simulink model "L_I"  (R2013a)
settings: Solver=ode45  StartTime=0.0  StopTime=0.2  RelTol=1e-3
settings Model: Creator=MEHEDI HASSAN  LastModifiedBy=MEHEDI HASSAN
settings OptimizationCC: InlineParams=on
settings DebuggingCC: SolverPrmCheckMsg=none  ModelReferenceExtraNoncontSigs=none

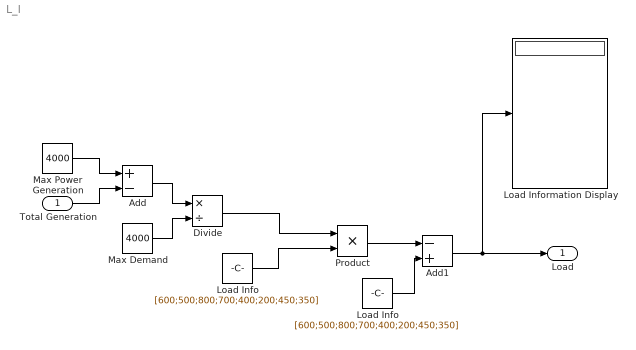
== system L_I ==
  Total Generation : Inport
  Add : Sum  Inputs=+-
  Add1 : Sum  Inputs=-+
  Divide : Product  Inputs=*/
  Load Info : Constant  Value=[600;500;800;700;400;200;450;350]
  "Load Info " : Constant  Value=[600;500;800;700;400;200;450;350]
  Load Information Display : Display
  Max Demand : Constant  Value=4000
  Max Power Generation : Constant  Value=4000
  Product : Product
  Load : Outport
  wires:
  Max Power Generation/1 -> Add/1
  Add/1 -> Divide/1
  Max Demand/1 -> Divide/2
  Divide/1 -> Product/1
  Load Info/1 -> Product/2
  Product/1 -> Add1/1
  "Load Info "/1 -> Add1/2
  Add1/1 -> Load/1, Load Information Display/1
  Total Generation/1 -> Add/2
